simulink model "blockDiagram"  (R2018b)
settings: Solver=VariableStepAuto  StartTime=0.0  StopTime=50  RelTol=1e-3
values from neighbouring files (symbols this model uses):
  Bd = 1    [matlab.mat]
  Kb = 0.00416666666667    [matlab.mat]
  Kd = 3    [matlab.mat]
  Kt = 0.0398    [matlab.mat]
  L = 0.000281    [matlab.mat]
  R = 1.45    [matlab.mat]
undefined symbols (not defined in the file or in its folder): theta
libraries: simulink x1
settings Model: Creator=holyCow  LastModifiedBy=holyCow

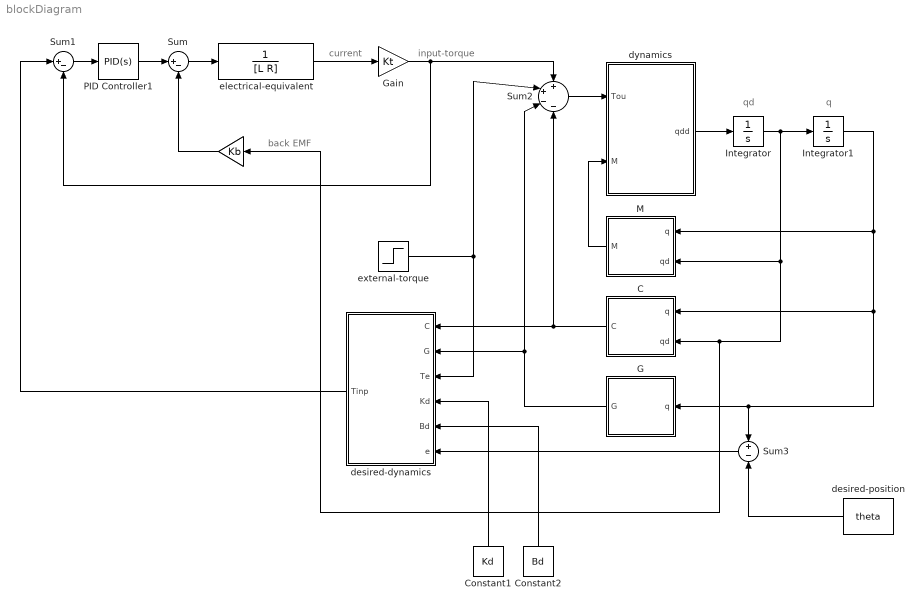
== system blockDiagram ==
  note: q
  note: qd
  note: back EMF
  note: current
  note: input-torque
  " " : Gain  Gain=Kb
  C : MATLAB Function  TreatAsAtomicUnit=on
  Constant1 : Constant  Value=Kd
  Constant2 : Constant  Value=Bd
  G : MATLAB Function  TreatAsAtomicUnit=on
  Gain : Gain  Gain=Kt
  Integrator : Integrator
  Integrator1 : Integrator
  M : MATLAB Function  TreatAsAtomicUnit=on
  PID Controller1 : simulink/Continuous/PID Controller  Controller=PID  Form=Parallel  TimeDomain=Continuous-time  SampleTime=-1  IntegratorMethod=Forward Euler  FilterMethod=Forward Euler  ControllerParametersSource=internal  P=0.00262223631261022  I=0.0812034556612777  D=0  UseFilter=on  N=100  TunerSelectOption=Transfer Function Based (PID Tuner App)  InitialConditionSource=internal  InitialConditionForIntegrator=0  InitialConditionForFilter=0  DifferentiatorICPrevScaledInput=0  ExternalReset=none  TrackingMode=off  Kt=1  LimitOutput=off  UpperSaturationLimit=inf  LowerSaturationLimit=-inf  LinearizeAsGain=on  AntiWindupMode=none  Kb=1  POutMin=[]  POutMax=[]  IOutMin=[]  IOutMax=[]  DOutMin=[]  DOutMax=[]  NOutMin=[]  NOutMax=[]  SumOutMin=[]  SumOutMax=[]  SaturationOutMin=[]  SaturationOutMax=[]  PParamMin=[]  PParamMax=[]  IParamMin=[]  IParamMax=[]  DParamMin=[]  DParamMax=[]  NParamMin=[]  NParamMax=[]  KbParamMin=[]  KbParamMax=[]  KtParamMin=[]  KtParamMax=[]  KbOutMin=[]  KbOutMax=[]  KtOutMin=[]  KtOutMax=[]  IntegratorOutMin=[]  IntegratorOutMax=[]  FilterOutMin=[]  FilterOutMax=[]  SumI1OutMin=[]  SumI1OutMax=[]  SumI2OutMin=[]  SumI2OutMax=[]  SumI3OutMin=[]  SumI3OutMax=[]  SumI4OutMin=[]  SumI4OutMax=[]  SumDOutMin=[]  SumDOutMax=[]  DifferentiatorOutMin=[]  DifferentiatorOutMax=[]  FilterDiffOutCoefMin=[]  FilterDiffOutCoefMax=[]  ReciprocalOutMin=[]  ReciprocalOutMax=[]  SumDenOutMin=[]  SumDenOutMax=[]  SumNumOutMin=[]  SumNumOutMax=[]  DivideOutMin=[]  DivideOutMax=[]  IntegratorContinuousStateAttributes=''  IntegratorStateMustResolveToSignalObject=off  IntegratorRTWStateStorageClass=Auto  FilterContinuousStateAttributes=''  FilterStateMustResolveToSignalObject=off  FilterRTWStateStorageClass=Auto  ParallelPVariant=InternalParameters  IdealPVariant=Disabled  IVariant=InternalParameters  DVariant=InternalParameters  IntegratorVariant=Continuous  SatVariant=Disabled  AWVariant=Passthrough  PCopyVariant=Disabled  TRVariant=Disabled  FdbkBlocksVariant=Forward  IdealPFdbkVariant=Disabled  SatFdbkVariant=Disabled  DerivativeFilterVariant=ContFilter  NVariant=InternalParameters  NCopyVariant=Disabled  FilterICVariant=InternalICsFilter  IntegratorICVariant=InternalICs  ExternalResetVariant=Disabled  TRSumVariant=Passthrough  SumFdbkVariant=Disabled  SumVariant=Sum_PID
  Sum : Sum  Inputs=|+-
  Sum1 : Sum  Inputs=|+-
  Sum2 : Sum  Inputs=++--
  Sum3 : Sum  Inputs=+-
  desired-dynamics : MATLAB Function  TreatAsAtomicUnit=on
  desired-position : Constant  Value=theta
  dynamics : MATLAB Function  TreatAsAtomicUnit=on
  electrical-equivalent : TransferFcn  Denominator=[L R]
  external-torque : Step  Time=5  After=0  SampleTime=0
  wires:
  Integrator1/1 -> M/1(q), G/1(q), Sum3/1, C/1(q)
  external-torque/1 -> Sum2/2, desired-dynamics/3(Te)
  desired-dynamics/1(Tinp) -> Sum1/1
  dynamics/1(qdd) -> Integrator/1
  " "/1 -> Sum/2
  PID Controller1/1 -> Sum/1
  electrical-equivalent/1 -> Gain/1
  Sum1/1 -> PID Controller1/1
  Sum/1 -> electrical-equivalent/1
  Integrator/1 -> Integrator1/1, " "/1, C/2(qd), M/2(qd)
  Gain/1 -> Sum2/1, Sum1/2
  M/1(M) -> dynamics/2(M)
  C/1(C) -> desired-dynamics/1(C), Sum2/4
  G/1(G) -> Sum2/3, desired-dynamics/2(G)
  Sum2/1 -> dynamics/1(Tou)
  desired-position/1 -> Sum3/2
  Sum3/1 -> desired-dynamics/6(e)
  Constant1/1 -> desired-dynamics/4(Kd)
  Constant2/1 -> desired-dynamics/5(Bd)

== matlab function blockDiagram/desired-dynamics ==
  data: C input; G input; Te input; Kd input; Bd input; Tinp output; e input
function Tinp = fcn(C, G, Te, Kd, Bd, e)
%params;
Kb = 0.1;
Kk = 0.2;

Tinp = Kb*C + Kk*G - Te;

== matlab function blockDiagram/M ==
  data: q input; M output; qd input
function M = fcn(q, qd)

M = qd;

== matlab function blockDiagram/C ==
  data: q input; C output; qd input
function C = fcn(q, qd)

C = qd;

== matlab function blockDiagram/G ==
  data: q input; G output
function G = fcn(q)

C = q;

== matlab function blockDiagram/dynamics ==
  data: Tou input; qdd output; M input
function qdd   = fcn(Tou, M)
l = 0.265;
m = 0.170;
a = 0.110;
b = 0.090;

g = 9.81;

m1 = 2.5;
m2 = 0.2;
mr = 0.1;
mf = 0.075;

% measure of radius
rr = 0.110/2;
rf = 0.075/2;

delta = rr - rf;

% l*sin(q2) + delta = m*sin(q1 - q2)
ta = (l/m + cos(q))^2 + (sin(q))^2;
tb = -2*(delta/m)*sin(q);
tc = (delta/m)^2 - (l/m + cos(q))^2;

q2 = acos((-tb + sqrt(tb^2 - 4*ta*tc))/(2*ta));
k = -1/(1 + ((l*cos(q2))/(m*cos(q - q2))));
%q2D = k * q1D;

x = sqrt(l^2 + m^2 - delta^2 + 2*l*m*cos(q));
c = ((-l*m*sin(q))/x);
%xD = c * q1D;

s = -1 * (l*k*m*sin(q2)*cos(q - q2) - l*m*cos(q2)*sin(q - q2)*(1 - k))/((l*cos(q2) + m*cos(q - q2))^2);
u = (l*m*(c*sin(q) - x*cos(q)))/(x^2);

%kD = s * q1D;
%cD = u * q1D;

%xa = a*cos(q2);
%xaD = -a*sin(q2)*q2D;

%ya = rr + a*sin(q2);
%yaD = a*cos(q2)*q2D;

%xb = x - b*cos(q - q2);
%xbD = xD + b*sin(q1 - q2)*(q1D - q2D);

%yb = rf + b*sin(q1 - q2);
%ybD = b*cos(q1 - q2)*(q1D - q2D);

%K = 0.5*m1*(xaD^2 + yaD^2) + 0.5*m2*(xbD^2 + ybD^2) + 0.75*mf*xD^2;
%P = mr*g*rr + mf*g*rf + m1*g*ya + m2*g*yb;

M = m1*(a^2)*(k^2) + (m2 + 1.5*mf)*(c^2) + m2*(b^2)*((1-k)^2) + 2*m2*b*sin(q - q2)*c*(1-k);

ctemp = cos(q - q2)*c*((1-k)^2) + sin(q - q2)*u*(1-k) - sin(q - q2)*c*s;
C = (m1*(a^2)*k*s + (m2 + 1.5*mf)*c*u - m2*(b^2)*s*(1-k) + m2*b*ctemp) * (qD^2);

G = m1*g*a*cos(q2)*k + m2*g*b*cos(q - q2)*(1 - k);

%N2 = (m1*g*xa + m2*g*xb)/(x);
%N1 = (((m1+m2)*x - m1*xa - m2*xb)*g)/(x);
%T_ext = Text + N1*l*cos(q2) - N2*m*cos(q1 - q2);
%Text = Fx*l*sin(q - q2) - Fy*m*cos(q - q2);
qdd = (Tou + Te - C - G)/M;
